simulink library "SimscapeCustomComponents_lib"  (R2025b)
settings: Solver=VariableStepAuto  StartTime=0.0  StopTime=10.0  RelTol=1e-3
undefined symbols (not defined in the file or in its folder): base, baseVdc, capacity, DiscIntNeverNeededParam, ee_sli_rtmsupport, filterInductance, freqeuncy, frequency, gcbh, gflInverter, gfmInverter, iMaxPU, Inertia, initialSOC, plantRating, solar, Ts, ups, Vac, windSystem, windTurbine
libraries: fl_lib x397, nesl_utility x171, eeGeneralControl x85, ee_lib x82, simulink x72, datacenter_lib x68, eeTransforms x38, slpidlib x24, buildingEnergy_lib x20, SimscapeFluids_lib x17, eeSinusoidalMeasurementV2 x8, eePwmGenerator x8
(part 18 of 24)

== system SimscapeCustomComponents_lib/Microgrid and Renewables/Sources/Wind Plant Integrated/Detailed/Wind Turbine and Converters/Wind Plant ==
  Pitch : Inport
  Wind speed : Inport  Port=2
  Chopper : Inport  Port=3
  Machine : Inport  Port=4
  Grid : Inport  Port=5
  Back-to-Back Converters : Subsystem  Variant=on  VariantControlMode=label  LabelModeActiveChoice=Switching  mask{converterFidelity=Switching, capDC=capDC, fSw=fSw}
      mask prompts: converterFidelity "Converter Fidelity"; capDC "DC bus capacitance (F)"; fSw "Switching Frequency (kHz)"
      settings: CopyFcn=set_param(gcb,'LinkStatus','none');
      mask TypeOptions converterFidelity: Average | Switching
      mask Callback converterFidelity: component.mask.converterFidelity(gcb);
      mask DialogControl editMSConverter Prompt: Edit machine  side converter parameters
      mask DialogControl editMSConverter Callback:
      | converterFidelity = get_param(gcb,'converterFidelity');
      | if strcmp(converterFidelity,'Average')
      |     blockPath = [gcb,'/',converterFidelity,'/','Machine Side Converter'];
      | else
      |     blockPath = [gcb,'/',converterFidelity,'/','Machine Side Converter','/','Converter'];
      | end
      |     component.mask.openConverterBlock(blockPath);
      mask DialogControl editGSConverter Prompt: Edit grid  side converter parameters
      mask DialogControl editGSConverter Callback:
      | converterFidelity = get_param(gcb,'converterFidelity');
      | if strcmp(converterFidelity,'Average')
      |     blockPath = [gcb,'/',converterFidelity,'/','Grid Side Converter'];
      | else
      |     blockPath = [gcb,'/',converterFidelity,'/','Grid Side Converter','/','Converter'];
      | end
      | component.mask.openConverterBlock(blockPath);
  Current Sensor (Three-Phase) : ee_lib/Sensors & Transducers/Current Sensor (Three-Phase)
  Ideal Torque Sensor : fl_lib/Mechanical/Mechanical Sensors/Ideal Torque Sensor
  Mechanical Rotational Reference2 : fl_lib/Mechanical/Rotational Elements/Mechanical Rotational Reference
  Mechanical Rotational Reference3 : fl_lib/Mechanical/Rotational Elements/Mechanical Rotational Reference
  PMSG : ee_lib/Electromechanical/Permanent Magnet/PMSM  port_option=ee.enum.threePhasePort.composite  winding_type=ee.enum.statorconnection.wye  machine_param=ee.enum.pmsm.parameterization.constant  nPolePairs=p  pmflux_param=ee.enum.pmflux.fluxlinkage  pm_flux_linkage=psim Wb  torque_constant=0.18 N*m/A  back_emf_constant=0.18 V*s/rad  stator_param=ee.enum.statorparam.LdLqL0  Ld=Ld H  Lq=Lq H  idVec=[-200, 0, 200] A  iqVec=[-200, 0, 200] A  LdMatrix=0.0002 * ones(3, 3) H  LqMatrix=0.0002 * ones(3, 3) H  PmMatrix=0.1 * ones(3, 3) Wb  ktMatrix=0.18 * ones(3, 3) N*m/A  keMatrix=0.18 * ones(3, 3) V*s/rad  L0=0.00016 H  Ls=0.0002 H  Lm=-0.00002 H  Ms=0.00002 H  Rs=Rs Ohm  zero_sequence=ee.enum.park.zerosequence.exclude  axes_param=ee.enum.rotorangle.qaxis  loss_param=ee.enum.ironloss.none  losses_oc=[0, 0, 0] W  losses_sc=[0, 0, 0] W  f_losses=60 Hz  Isc_losses=95 A  J=200 kg*m^2  lam=1e-2 N*m*s/rad  i_d_specify=off  i_d_priority=None  i_d=0 A  i_d_nominal_specify=off  i_d_nominal_value=1  i_d_nominal_unit=A  i_q_specify=off  i_q_priority=None  i_q=0 A  i_q_nominal_specify=off  i_q_nominal_value=1  i_q_nominal_unit=A  torque_specify=off  torque_priority=None  torque=0 N*m  torque_nominal_specify=off  torque_nominal_value=1  torque_nominal_unit=N*m  angular_velocity_specify=off  angular_velocity_priority=Low  angular_velocity=2.26 rad/s  angular_velocity_nominal_specify=off  angular_velocity_nominal_value=1  angular_velocity_nominal_unit=rpm  angular_position_specify=off  angular_position_priority=High  angular_position=0 deg  angular_position_nominal_specify=off  angular_position_nominal_value=1  angular_position_nominal_unit=deg  alpha=3.93e-3 1/K  alpha_flux=-0.001 1/K  Tmeas=298.15 K  stator_thermal_mass=100 J/K  rotor_thermal_mass=200 J/K  Rm_percent_rotor=90  Rd_percent_rotor=30  temperatureA_specify=off  temperatureA_priority=High  temperatureA=25 degC  temperatureA_nominal_specify=off  temperatureA_nominal_value=1  temperatureA_nominal_unit=degC  temperatureB_specify=off  temperatureB_priority=High  temperatureB=25 degC  temperatureB_nominal_specify=off  temperatureB_nominal_value=1  temperatureB_nominal_unit=degC  temperatureC_specify=off  temperatureC_priority=High  temperatureC=25 degC  temperatureC_nominal_specify=off  temperatureC_nominal_value=1  temperatureC_nominal_unit=degC  temperatureR_specify=off  temperatureR_priority=High  temperatureR=25 degC  temperatureR_nominal_specify=off  temperatureR_nominal_value=1  temperatureR_nominal_unit=degC
      settings: InternalSimscapePortConfiguration="{\"Bottom\":[],\"Left\":[{\"id\":\"N\",\"label\":\"~\",\"type\":\"foundation.electrical.three_phase\"}],\"Right\":[{\"id\":\"R\",\"label\":\"R\",\"type\":\"foundation.mechanical.rotational.rotational\"},{\"id\":\"C\",\"label\":\"C\",\"type\":\"foundation.mechanical.rotational.rotational\"}],\"Top\":[]}"
  PS-Simulink Converter : nesl_utility/PS-Simulink Converter  PhysicalDomain=network_engine_domain  SubClassName=ps_output  LeftPortType=input  RightPortType=output  PseudoPeriodic=off  Frequencies=[]  VectorFormat=1-D array  Unit=A  AffineConversion=off
  PS-Simulink Converter1 : nesl_utility/PS-Simulink Converter  PhysicalDomain=network_engine_domain  SubClassName=ps_output  LeftPortType=input  RightPortType=output  PseudoPeriodic=off  Frequencies=[]  VectorFormat=inherit  Unit=rad/s  AffineConversion=off
  PS-Simulink Converter5 : nesl_utility/PS-Simulink Converter  PhysicalDomain=network_engine_domain  SubClassName=ps_output  LeftPortType=input  RightPortType=output  PseudoPeriodic=off  Frequencies=[]  VectorFormat=1-D array  Unit=N*m  AffineConversion=off
  PS-Simulink Converter7 : nesl_utility/PS-Simulink Converter  PhysicalDomain=network_engine_domain  SubClassName=ps_output  LeftPortType=input  RightPortType=output  PseudoPeriodic=off  Frequencies=[]  VectorFormat=1-D array  Unit=rad  AffineConversion=off
  Rotational Motion Sensor : fl_lib/Mechanical/Mechanical Sensors/Ideal Rotational Motion Sensor  reference=foundation.enum.MeasurementReference.difference  acceleration_port=false  velocity_port=true  position_port=true  wrap_angle=simscape.enum.onoff.off  offset=0 deg
  Scope1 : Scope
      settings: ActiveDisplayYMinimum=-6255.05498425373  ActiveDisplayYMaximum=6362.825931701329  DataLoggingVariableName=ScopeData6
  Simulink-PS Converter : nesl_utility/Simulink-PS Converter  PhysicalDomain=network_engine_domain  SubClassName=ps_input  LeftPortType=input  RightPortType=output  PseudoPeriodic=off  Frequencies=[]  NoiseDistribution=none  NoiseParameters=[]  Unit=1  AffineConversion=off  FilteringAndDerivatives=provide  SimscapeFilterOrder=1  InputFilterTimeConstant=0.001  UdotUserProvided=0
  Simulink-PS Converter1 : nesl_utility/Simulink-PS Converter  PhysicalDomain=network_engine_domain  SubClassName=ps_input  LeftPortType=input  RightPortType=output  PseudoPeriodic=off  Frequencies=[]  NoiseDistribution=none  NoiseParameters=[]  Unit=1  AffineConversion=off  FilteringAndDerivatives=provide  SimscapeFilterOrder=1  InputFilterTimeConstant=0.001  UdotUserProvided=0
  Unit Delay : UnitDelay  SampleTime=-1
  Wind Turbine : ee_lib/Electromechanical/Wind Turbine (Mechanical)  R_rotor=turbineRadius m  pitch_TLU=pitch deg  lambda_TLU=TSR  Cp_TLU=cp  v_thr=wt m/s  w_thr=rt rad/s  rho_air=airDensity kg/m^3  includeInertia=false  J=Inertia kg*m^2  lam=10 N*m*s/rad  w_specify=off  w_priority=Low  w=2.262*2.5 rad/s  w_nominal_specify=off  w_nominal_value=1  w_nominal_unit=rad/s  t_specify=off  t_priority=None  t=0 N*m  t_nominal_specify=off  t_nominal_value=1  t_nominal_unit=N*m  Torque_specify=off  Torque_priority=None  Torque=0 N*m  Torque_nominal_specify=off  Torque_nominal_value=1  Torque_nominal_unit=N*m
      settings: InternalSimscapePortConfiguration="{\"Bottom\":[],\"Left\":[{\"id\":\"vWind\",\"label\":\"V\",\"type\":\"input\"},{\"id\":\"pitch\",\"label\":\"β\",\"type\":\"input\"}],\"Right\":[{\"id\":\"R\",\"label\":\"R\",\"type\":\"foundation.mechanical.rotational.rotational\"}],\"Top\":[]}"
  ~ : PMIOPort  Side=Right
  Out Bus Element2 : Outport  PortName=PMSM  Element=torque
  Out Bus Element3 : Outport  PortName=PMSM  Element=rotorSpeed
  BusElementOut : Outport  PortName=PMSM  Element=rotorAngle
  BusElementOut1 : Outport  PortName=PMSM  Element=iabc
  Out Bus Element : Outport  Port=2  PortName=Meas  Element=windSpeed
  BusElementOut2 : Outport  Port=2  PortName=Meas  Element=Vdc
  wires:
  PS-Simulink Converter7/1 -> BusElementOut/1
  Grid/1 -> Back-to-Back Converters/3(Grid_ref)
  Chopper/1 -> Back-to-Back Converters/1(Chopper)
  PS-Simulink Converter1/1 -> Out Bus Element3/1
  Pitch/1 -> Simulink-PS Converter/1
  Unit Delay/1 -> Out Bus Element/1
  PS-Simulink Converter/1 -> Scope1/1, BusElementOut1/1
  Wind speed/1 -> Unit Delay/1, Simulink-PS Converter1/1
  PS-Simulink Converter5/1 -> Out Bus Element2/1
  Machine/1 -> Back-to-Back Converters/2(SM_ref)
  Back-to-Back Converters/1(Vdc) -> BusElementOut2/1
  connections:
  Current Sensor (Three-Phase)/RConn1 -- PS-Simulink Converter/LConn1
  Back-to-Back Converters/RConn1 -- ~/RConn1
  PS-Simulink Converter7/LConn1 -- Rotational Motion Sensor/RConn3
  PS-Simulink Converter1/LConn1 -- Rotational Motion Sensor/RConn2
  Current Sensor (Three-Phase)/LConn1 -- PMSG/LConn1
  PMSG/RConn2 -- Mechanical Rotational Reference2/LConn1
  Ideal Torque Sensor/RConn1 -- Wind Turbine/RConn1 -- Rotational Motion Sensor/LConn1
  PMSG/RConn1 -- Ideal Torque Sensor/LConn1
  Mechanical Rotational Reference3/LConn1 -- Rotational Motion Sensor/RConn1
  PS-Simulink Converter5/LConn1 -- Ideal Torque Sensor/RConn2
  Current Sensor (Three-Phase)/RConn2 -- Back-to-Back Converters/LConn1
  Wind Turbine/LConn2 -- Simulink-PS Converter/RConn1
  Wind Turbine/LConn1 -- Simulink-PS Converter1/RConn1

== system SimscapeCustomComponents_lib/Microgrid and Renewables/Storage/BESS Integrated/Detailed/BESS Controller/Grid Following ==
  VRef : Inport
  FRef : Inport  Port=2
  PRef : Inport  Port=3
  QRef : Inport  Port=4
  Mode : Inport  Port=5
  Reset : Inport  Port=6
  In Bus Element3 : Inport  Port=7  PortName=VIBus  Element=Vd
  BusElementIn : Inport  Port=7  PortName=VIBus  Element=Vd
  In Bus Element2 : Inport  Port=7  PortName=VIBus  Element=Vq
  In Bus Element7 : Inport  Port=7  PortName=VIBus  Element=Theta
  BusElementIn1 : Inport  Port=7  PortName=VIBus  Element=Freq
  BusElementIn3 : Inport  Port=7  PortName=VIBus  Element=Id
  BusElementIn4 : Inport  Port=7  PortName=VIBus  Element=Iq
  Constant : Constant  Value=10
  Current_controller : Subsystem
  Inverse Park Transform1 : eeTransforms/Inverse Park Transform  AxisAlignment=Q-axis  PowerInvariant=off
  Reference Current : Subsystem
  Sum2 : Sum  Inputs=|+-
  Terminator : Terminator
  Terminator1 : Terminator
  Unit Delay : UnitDelay  SampleTime=Td
  Unit Delay1 : UnitDelay  SampleTime=Td
  Unit Delay2 : UnitDelay  SampleTime=Ts
  mabc : Outport
  wires:
  Constant/1 -> Reference Current/4(LVRT_iq)
  Reset/1 -> Terminator1/1
  Mode/1 -> Terminator/1
  In Bus Element2/1 -> Current_controller/6(Vq)
  Inverse Park Transform1/1 -> Unit Delay2/1
  Unit Delay2/1 -> mabc/1
  Current_controller/1(mdq0) -> Inverse Park Transform1/1
  In Bus Element3/1 -> Current_controller/5(Vd)
  In Bus Element7/1 -> Inverse Park Transform1/2
  FRef/1 -> Sum2/1
  VRef/1 -> Reference Current/1(V_ref)
  Sum2/1 -> Reference Current/3(del f)
  Reference Current/2(iq_ref) -> Current_controller/3(iqref)
  Reference Current/1(id_ref) -> Current_controller/1(id-ref)
  Unit Delay1/1 -> Sum2/2
  Unit Delay/1 -> Reference Current/2(V-mag)
  BusElementIn/1 -> Unit Delay/1
  BusElementIn1/1 -> Unit Delay1/1
  BusElementIn3/1 -> Current_controller/2(ipvd)
  BusElementIn4/1 -> Current_controller/4(iq)
  PRef/1 -> Reference Current/5(PRef)
  QRef/1 -> Reference Current/6(QRef)

== system SimscapeCustomComponents_lib/Microgrid and Renewables/Storage/BESS Integrated/Detailed/BESS Controller/Grid Forming ==
  VRef : Inport
  FRef : Inport  Port=2
  PRef : Inport  Port=3
  QRef : Inport  Port=4
  Mode : Inport  Port=5
  Reset : Inport  Port=6
  Bus Element In : Inport  Port=7  PortName=VIBus  Element=Vabc
  BusElementIn : Inport  Port=7  PortName=VIBus  Element=Iabc
  Current Limiting : Subsystem
  Grid Voltage Reactive Power Support : Subsystem
  Measurement : Subsystem
      mask Display: image('meas2_1_7_7_2_1.png');
  Power Control : Subsystem
  Subsystem2 : Subsystem
      settings: PortSchema="{\"entries\":[{\"content\":{\"sides\":[{\"content\":{\"connectorIds\":[\"Out1\"]},\"type\":\"ConnectorPlacement.EquallySpacedRectSide\",\"uuid\":\"7526c1f7-0aba-4355-8bbd-47d168879ecb\"},{\"content\":{\"connectorIds\":[\"In1\",\"In2\"],\"side\":\"RIGHT\"},\"type\":\"ConnectorPlacement.EquallySpacedRectSide\",\"uuid\":\"1dda9693-ec76-4df0-8ad4-aaa83d2574b3\"},{\"content\":{\"side\":\"TOP\"},\"type\":\"ConnectorPlacement.EquallySpacedRectSide\",\"uuid\":\"71ea411b-eb5f-4279-ae23-08ebb3ff1ed6\"}]},\"type\":\"ConnectorPlacement.EquallySpacedConnector\",\"uuid\":\"19864e0c-0998-460d-9705-13c69283d4ec\"}],\"packageUris\":[\"http://schema.mathworks.com/mf0/Connector/R2020b\"],\"version\":\"1.0\"}"
  Terminator : Terminator
  Terminator1 : Terminator
  Terminator2 : Terminator
  VoltageCurrentControl : Subsystem
      settings: PortSchema="{\"entries\":[{\"content\":{\"sides\":[{\"content\":{\"connectorIds\":[\"In1\",\"In2\",\"In3\"]},\"type\":\"ConnectorPlacement.EquallySpacedRectSide\",\"uuid\":\"0bf15a12-7bc0-47e4-89bd-435769673763\"},{\"content\":{\"connectorIds\":[\"Out1\"],\"side\":\"RIGHT\"},\"type\":\"ConnectorPlacement.EquallySpacedRectSide\",\"uuid\":\"44a15d74-8878-4ec6-abe4-be0b1b609519\"},{\"content\":{\"connectorIds\":[\"In4\"],\"side\":\"TOP\"},\"type\":\"ConnectorPlacement.EquallySpacedRectSide\",\"uuid\":\"7a96781e-5638-4b2a-8101-d5785aae9f0f\"}]},\"type\":\"ConnectorPlacement.EquallySpacedConnector\",\"uuid\":\"4b3373ad-cf20-4175-894e-3bd1604dd0ce\"}],\"packageUris\":[\"http://schema.mathworks.com/mf0/Connector/R2020b\"],\"version\":\"1.0\"}"
  mabc : Outport
  wires:
  Subsystem2/1(mabc) -> mabc/1
  VoltageCurrentControl/1(mabc) -> Subsystem2/1(In)
  Bus Element In/1 -> Measurement/1(Vgabcc)
  BusElementIn/1 -> Measurement/2(Igabc)
  Measurement/2(Pmeas) -> Terminator/1
  Measurement/3(Qmeas) -> Terminator1/1
  Measurement/1(measure) -> Current Limiting/1(measure), VoltageCurrentControl/4(measure), Power Control/1(measure), Grid Voltage Reactive Power Support/1(measure)
  Power Control/3(angle) -> Measurement/3(Angle)
  Power Control/1(reactiveControl) -> Current Limiting/2(reactiveControl)
  Power Control/2(activeControl) -> VoltageCurrentControl/2(activeControl)
  Current Limiting/1(currentLimiting) -> VoltageCurrentControl/1(currentLimiting)
  QRef/1 -> Grid Voltage Reactive Power Support/3(QrefInput)
  PRef/1 -> Grid Voltage Reactive Power Support/2(PrefInput)
  Grid Voltage Reactive Power Support/1(Pref) -> Power Control/2(Pref)
  Grid Voltage Reactive Power Support/2(Qref) -> Power Control/3(Qref)
  Measurement/4(fmeas) -> Terminator2/1
  FRef/1 -> Power Control/5(Fref)
  VRef/1 -> Power Control/4(Vref)
  Mode/1 -> Power Control/6(CntrlFlag)
  Reset/1 -> VoltageCurrentControl/3(Reset), Subsystem2/2(Reset)

== system SimscapeCustomComponents_lib/Microgrid and Renewables/Storage/BESS Integrated/Detailed/BESS Plant/Converter ==
  mabc : Inport
  Average : Subsystem  VariantControl=Average
  Switching : Subsystem  VariantControl=Switching
  + : PMIOPort  Side=Left
  - : PMIOPort  Port=2  Side=Left
  ~ : PMIOPort  Port=3  Side=Right

== system SimscapeCustomComponents_lib/Microgrid and Renewables/Storage/BESS Integrated/Detailed/Filter & Measurements/PLL & Measurements ==
  V : Inport
  I : Inport  Port=2
  Measurement1 : Subsystem
  Measurement2 : Subsystem
  Subsystem : Subsystem
  Out Bus Element : Outport  PortName=VIbus  Element=Vq
  Out Bus Element1 : Outport  PortName=VIbus  Element=Vd
  Out Bus Element2 : Outport  PortName=VIbus  Element=Freq
  Out Bus Element3 : Outport  PortName=VIbus  Element=Theta
  Out Bus Element4 : Outport  PortName=VIbus  Element=Vmag
  Out Bus Element5 : Outport  PortName=VIbus  Element=Iq
  Out Bus Element6 : Outport  PortName=VIbus  Element=Id
  Out Bus Element7 : Outport  PortName=VIbus  Element=Iabc
  Out Bus Element8 : Outport  PortName=VIbus  Element=Vabc
  wires:
  V/1 -> Measurement2/1(u)
  Subsystem/2(freq) -> Out Bus Element2/1
  Subsystem/5(Vq) -> Out Bus Element/1
  Subsystem/3(angle) -> Out Bus Element3/1
  Subsystem/4(Vd) -> Out Bus Element1/1
  Measurement2/1(Vg) -> Out Bus Element8/1, Subsystem/1(Vabc)
  Subsystem/1(mag) -> Out Bus Element4/1
  I/1 -> Measurement1/1(u)
  Measurement1/1(Vg) -> Out Bus Element7/1, Subsystem/2(Iabc)
  Subsystem/7(Iq1) -> Out Bus Element5/1
  Subsystem/6(Id1) -> Out Bus Element6/1

== system SimscapeCustomComponents_lib/Microgrid and Renewables/Storage/BESS Integrated/Simplified/Grid Following/Measurements ==
  Current and Voltage Sensor (Three-Phase)1 : ee_lib/Sensors & Transducers/Current and Voltage Sensor (Three-Phase)  vMeasurementType=ee.enum.vmeasurement.lg  outputUnit=ee.enum.unit.pu  SRated=plantRating*1000 A*V  VRated=Vac V  I_specify=off  I_priority=None  I=[0, 0, 0] A  I_nominal_specify=off  I_nominal_value=1  I_nominal_unit=A  V_specify=off  V_priority=None  V=[0, 0, 0] V  V_nominal_specify=off  V_nominal_value=1  V_nominal_unit=V
      settings: InternalSimscapePortConfiguration="{\"Bottom\":[],\"Left\":[{\"id\":\"N1\",\"label\":\"~1\",\"type\":\"foundation.electrical.three_phase\"}],\"Right\":[{\"id\":\"V_output\",\"label\":\"V\",\"type\":\"output\"},{\"id\":\"I_output\",\"label\":\"I\",\"type\":\"output\"},{\"id\":\"N2\",\"label\":\"~2\",\"type\":\"foundation.electrical.three_phase\"}],\"Top\":[]}"
  Gain1 : Gain  Gain=1/(plantRating*1000)
  Gain2 : Gain  Gain=1/(plantRating*1000)
  Low-Pass Filter (Discrete or Continuous)1 : eeGeneralControl/Low-Pass Filter (Discrete or Continuous)  K=1  T=0.1  B=inf  A=-inf  init_option=Inherited from block input  x0=0  Ts=-1
  Low-Pass Filter (Discrete or Continuous)2 : eeGeneralControl/Low-Pass Filter (Discrete or Continuous)  K=1  T=0.1  B=inf  A=-inf  init_option=Inherited from block input  x0=0  Ts=-1
  PS-Simulink Converter{,1..3} (4 alike) : nesl_utility/PS-Simulink Converter  PhysicalDomain=network_engine_domain  SubClassName=ps_output  LeftPortType=input  RightPortType=output  PseudoPeriodic=off  Frequencies=[]  VectorFormat=inherit  Unit=inherit  AffineConversion=off
  Power Sensor (Three-Phase) : ee_lib/Sensors & Transducers/Power Sensor (Three-Phase)  load_type=ee.enum.passive.type_balanced.balanced  f0=60 Hz
      settings: InternalSimscapePortConfiguration="{\"Bottom\":[],\"Left\":[{\"id\":\"N1\",\"label\":\"~1\",\"type\":\"foundation.electrical.three_phase\"}],\"Right\":[{\"id\":\"N2\",\"label\":\"~2\",\"type\":\"foundation.electrical.three_phase\"}],\"Top\":[{\"id\":\"Pm\",\"label\":\"P\",\"type\":\"output\"},{\"id\":\"Qm\",\"label\":\"Q\",\"type\":\"output\"}]}"
  In : PMIOPort  Side=Left
  ~ : PMIOPort  Port=2  Side=Right
  P : Outport
  Q : Outport  Port=2
  V : Outport  Port=3
  I : Outport  Port=4
  wires:
  PS-Simulink Converter/1 -> Low-Pass Filter (Discrete or Continuous)1/1
  PS-Simulink Converter1/1 -> Low-Pass Filter (Discrete or Continuous)2/1
  Low-Pass Filter (Discrete or Continuous)1/1 -> Gain1/1
  Low-Pass Filter (Discrete or Continuous)2/1 -> Gain2/1
  PS-Simulink Converter2/1 -> V/1
  PS-Simulink Converter3/1 -> I/1
  Gain1/1 -> P/1
  Gain2/1 -> Q/1
  connections:
  Current and Voltage Sensor (Three-Phase)1/RConn1 -- PS-Simulink Converter2/LConn1
  PS-Simulink Converter/LConn1 -- Power Sensor (Three-Phase)/LConn2
  In/RConn1 -- Power Sensor (Three-Phase)/LConn1
  Current and Voltage Sensor (Three-Phase)1/RConn3 -- ~/RConn1
  PS-Simulink Converter1/LConn1 -- Power Sensor (Three-Phase)/LConn3
  Current and Voltage Sensor (Three-Phase)1/LConn1 -- Power Sensor (Three-Phase)/RConn1
  Current and Voltage Sensor (Three-Phase)1/RConn2 -- PS-Simulink Converter3/LConn1

== system SimscapeCustomComponents_lib/Microgrid and Renewables/Storage/BESS Integrated/Simplified/Grid Following/Power Limiter ==
  P : Inport
  SOC : Inport  Port=2
  V : Inport  Port=3
  Add : Sum
  Compare To Constant : simulink/Logic and Bit Operations/Compare To Constant  relop=<=  const=minSOC  OutDataTypeStr=boolean
  Compare To Constant1 : simulink/Logic and Bit Operations/Compare To Constant  relop=>=  const=maxSOC  OutDataTypeStr=boolean
  Constant : Constant  Value=maxSOC
  Constant1 : Constant  Value=0
  Constant2 : Constant  Value=minSOC
  Constant3 : Constant  Value=0
  Constant5 : Constant  Value=minSOC
  Data Type Conversion : DataTypeConversion  OutDataTypeStr=double  SaturateOnIntegerOverflow=off  RndMeth=Floor
  Delay1 : Delay  DelayLength=1
  Divide : Product  Inputs=*/
  Gain : Gain  Gain=-1/(Inf)
  GreaterThan : RelationalOperator  Operator=>  OutDataTypeStr=boolean  RndMeth=Simplest  InputSameDT=off
  GreaterThan1 : RelationalOperator  Operator=<  OutDataTypeStr=boolean  RndMeth=Simplest  InputSameDT=off
  GreaterThan3 : RelationalOperator  Operator=<  OutDataTypeStr=boolean  RndMeth=Simplest  InputSameDT=off
  NOR : Logic  Operator=NOR  IconShape=distinctive  AllPortsSameDT=off  OutDataTypeStr=boolean
  Product : Product
  Scope1 : Scope  NumInputPorts=2
  Scope2 : Scope
  Scope3 : Scope  NumInputPorts=3
  Switch : Switch  Criteria=u2 > Threshold  SaturateOnIntegerOverflow=off  InputSameDT=off
  Switch1 : Switch  Criteria=u2 > Threshold  SaturateOnIntegerOverflow=off  InputSameDT=off
  Switch2 : Switch  Criteria=u2 > Threshold  SaturateOnIntegerOverflow=off  InputSameDT=off
  POut : Outport
  SOCFlag : Outport  Port=2
  wires:
  P/1 -> Scope3/2, Switch2/2, Switch1/3, Switch/3
  Switch1/1 -> Scope3/1, Switch2/1
  Constant3/1 -> Switch1/1
  GreaterThan1/1 -> Scope1/1, Switch1/2
  Constant2/1 -> GreaterThan1/2
  Constant1/1 -> Switch/1
  GreaterThan/1 -> Switch/2
  Constant/1 -> GreaterThan/2
  Constant5/1 -> GreaterThan3/2
  GreaterThan3/1 -> SOCFlag/1
  V/1 -> Delay1/1
  Delay1/1 -> Divide/2
  Divide/1 -> Gain/1
  SOC/1 -> Add/2, GreaterThan3/1, Scope2/1, GreaterThan1/1, GreaterThan/1
  Switch/1 -> Scope3/3, Switch2/3
  Switch2/1 -> Divide/1, Product/1
  Add/1 -> Compare To Constant/1, Compare To Constant1/1
  Compare To Constant/1 -> NOR/1
  Compare To Constant1/1 -> NOR/2
  NOR/1 -> Data Type Conversion/1
  Data Type Conversion/1 -> Product/2
  Gain/1 -> Add/1
  Product/1 -> POut/1

== system SimscapeCustomComponents_lib/Microgrid and Renewables/Storage/BESS Integrated/Simplified/Grid Following/SOC Estimation ==
  I : Inport
  Constant : Constant  Value=0.95
  Gain : Gain  Gain=-1/(100000)
  Integrator (Discrete or Continuous) : eeGeneralControl/Integrator (Discrete or Continuous)  LabelModeActiveChoice=Discrete  IntegratorMethod=Integration: Forward Euler  ExternalReset=level  LimitType=Anti-windup  B=inf  A=-inf  Ts=-1
  SOC : Outport
  wires:
  Constant/1 -> Integrator (Discrete or Continuous)/3
  I/1 -> Gain/1
  Gain/1 -> Integrator (Discrete or Continuous)/1
  Integrator (Discrete or Continuous)/1 -> SOC/1

== system SimscapeCustomComponents_lib/Microgrid and Renewables/Storage/BESS Integrated/Simplified/Grid Forming/Limiter ==
  SOC : Inport
  Compare To Constant : simulink/Logic and Bit Operations/Compare To Constant  relop=<=  const=minSOC  OutDataTypeStr=boolean
  Compare To Constant1 : simulink/Logic and Bit Operations/Compare To Constant  relop=>=  const=maxSOC  OutDataTypeStr=boolean
  Data Type Conversion : DataTypeConversion  OutDataTypeStr=double  SaturateOnIntegerOverflow=off  RndMeth=Floor
  Delay : Delay  DelayLength=1  InputProcessing=Columns as channels (frame based)
  OR : Logic  Operator=OR  AllPortsSameDT=off  OutDataTypeStr=boolean
  Flag : Outport
  wires:
  SOC/1 -> Compare To Constant/1, Compare To Constant1/1
  Compare To Constant/1 -> OR/1
  Compare To Constant1/1 -> OR/2
  OR/1 -> Data Type Conversion/1
  Data Type Conversion/1 -> Delay/1
  Delay/1 -> Flag/1

== system SimscapeCustomComponents_lib/Microgrid and Renewables/Storage/BESS Integrated/Simplified/Grid Forming/Measurements ==
  Current and Voltage Sensor (Three-Phase)1 : ee_lib/Sensors & Transducers/Current and Voltage Sensor (Three-Phase)  vMeasurementType=ee.enum.vmeasurement.lg  outputUnit=ee.enum.unit.pu  SRated=plantRating*1000 A*V  VRated=Vac V  I_specify=off  I_priority=None  I=[0, 0, 0] A  I_nominal_specify=off  I_nominal_value=1  I_nominal_unit=A  V_specify=off  V_priority=None  V=[0, 0, 0] V  V_nominal_specify=off  V_nominal_value=1  V_nominal_unit=V
      settings: InternalSimscapePortConfiguration="{\"Bottom\":[],\"Left\":[{\"id\":\"N1\",\"label\":\"~1\",\"type\":\"foundation.electrical.three_phase\"}],\"Right\":[{\"id\":\"V_output\",\"label\":\"V\",\"type\":\"output\"},{\"id\":\"I_output\",\"label\":\"I\",\"type\":\"output\"},{\"id\":\"N2\",\"label\":\"~2\",\"type\":\"foundation.electrical.three_phase\"}],\"Top\":[]}"
  Gain1 : Gain  Gain=1/(plantRating*1000)
  Gain2 : Gain  Gain=1/(plantRating*1000)
  PS-Simulink Converter{,1..3} (4 alike) : nesl_utility/PS-Simulink Converter  PhysicalDomain=network_engine_domain  SubClassName=ps_output  LeftPortType=input  RightPortType=output  PseudoPeriodic=off  Frequencies=[]  VectorFormat=inherit  Unit=inherit  AffineConversion=off
  Power Sensor (Three-Phase) : ee_lib/Sensors & Transducers/Power Sensor (Three-Phase)  load_type=ee.enum.passive.type_balanced.balanced  f0=60 Hz
      settings: InternalSimscapePortConfiguration="{\"Bottom\":[],\"Left\":[{\"id\":\"N1\",\"label\":\"~1\",\"type\":\"foundation.electrical.three_phase\"}],\"Right\":[{\"id\":\"N2\",\"label\":\"~2\",\"type\":\"foundation.electrical.three_phase\"}],\"Top\":[{\"id\":\"Pm\",\"label\":\"P\",\"type\":\"output\"},{\"id\":\"Qm\",\"label\":\"Q\",\"type\":\"output\"}]}"
  In : PMIOPort  Side=Left
  ~ : PMIOPort  Port=2  Side=Right
  P : Outport
  Q : Outport  Port=2
  V : Outport  Port=3
  I : Outport  Port=4
  wires:
  Gain2/1 -> Q/1
  Gain1/1 -> P/1
  PS-Simulink Converter3/1 -> I/1
  PS-Simulink Converter2/1 -> V/1
  PS-Simulink Converter/1 -> Gain1/1
  PS-Simulink Converter1/1 -> Gain2/1
  connections:
  Current and Voltage Sensor (Three-Phase)1/RConn2 -- PS-Simulink Converter3/LConn1
  Current and Voltage Sensor (Three-Phase)1/LConn1 -- Power Sensor (Three-Phase)/RConn1
  PS-Simulink Converter1/LConn1 -- Power Sensor (Three-Phase)/LConn3
  Current and Voltage Sensor (Three-Phase)1/RConn3 -- ~/RConn1
  In/RConn1 -- Power Sensor (Three-Phase)/LConn1
  PS-Simulink Converter/LConn1 -- Power Sensor (Three-Phase)/LConn2
  Current and Voltage Sensor (Three-Phase)1/RConn1 -- PS-Simulink Converter2/LConn1

== system SimscapeCustomComponents_lib/Microgrid and Renewables/Storage/BESS Integrated/Simplified/Grid Forming/Reference Generator ==
  Mode : Inport
  PRef : Inport  Port=2
  P : Inport  Port=3
  QRef : Inport  Port=4
  Q : Inport  Port=5
  VRef : Inport  Port=6
  V : Inport  Port=7
  Gain : Gain  Gain=efficiency/100
  Gain2 : Gain  Gain=sqrt(3)/Vac
  If : If
  If Action Subsystem : Subsystem  TreatAsAtomicUnit=on
  If Action Subsystem1 : Subsystem  TreatAsAtomicUnit=on
  Merge : Merge
  Merge1 : Merge
  Vt : Outport
  Ph : Outport  Port=2
  wires:
  Merge/1 -> Vt/1
  Gain2/1 -> If Action Subsystem1/4(V)
  Q/1 -> If Action Subsystem/4(Q)
  P/1 -> If Action Subsystem1/2(P), If Action Subsystem/2(P)
  Merge1/1 -> Ph/1
  If Action Subsystem1/2(Ph) -> Merge1/2
  If Action Subsystem/2(Ph) -> Merge1/1
  If Action Subsystem1/1(Vt) -> Merge/2
  If Action Subsystem/1(Vt) -> Merge/1
  If/2 -> If Action Subsystem1/Action
  V/1 -> Gain2/1
  VRef/1 -> If Action Subsystem1/3(VRef)
  QRef/1 -> If Action Subsystem/3(QRef)
  PRef/1 -> If Action Subsystem1/1(PRef), Gain/1
  If/1 -> If Action Subsystem/Action
  Mode/1 -> If/1
  Gain/1 -> If Action Subsystem/1(PRef)

== system SimscapeCustomComponents_lib/Microgrid and Renewables/Storage/BESS Integrated/Simplified/Grid Forming/SOC Estimation ==
  P : Inport
  Constant : Constant  Value=Vdc
  Constant1 : Constant  Value=initialSOC
  Constant2 : Constant  Value=capacity
  Constant3 : Constant  Value=Inf
  Divide : Product  Inputs=*/
  Divide1 : Product  Inputs=*/
  Gain : Gain  Gain=-plantRating*1000
  Integrator (Discrete or Continuous) : eeGeneralControl/Integrator (Discrete or Continuous)  LabelModeActiveChoice=Discrete  IntegratorMethod=Integration: Forward Euler  ExternalReset=level  LimitType=Anti-windup  B=inf  A=-inf  Ts=-1
  String Compare : StringCompare
  String Constant : StringConstant  String=capacityType
  String Constant1 : StringConstant  String="\"Fixed\""
  Switch : Switch  Criteria=u2 > Threshold  SaturateOnIntegerOverflow=off  InputSameDT=off
  Meas : Outport
  wires:
  Constant3/1 -> Switch/3
  Constant2/1 -> Switch/1
  Divide1/1 -> Integrator (Discrete or Continuous)/1
  Switch/1 -> Divide1/2
  String Compare/1 -> Switch/2
  String Constant1/1 -> String Compare/2
  String Constant/1 -> String Compare/1
  Integrator (Discrete or Continuous)/1 -> Meas/1
  Constant1/1 -> Integrator (Discrete or Continuous)/3
  Divide/1 -> Divide1/1
  Constant/1 -> Divide/2
  P/1 -> Gain/1
  Gain/1 -> Divide/1

== system SimscapeCustomComponents_lib/Microgrid and Renewables/Storage/BESS Plant/Converter/Switching/Pulse Generation ==
  G : Inport
  Constant : Constant  Value=5
  Subtract : Sum  Inputs=-+
  G1 : Outport  VectorParamsAs1DForOutWhenUnconnected=off
  G2 : Outport  Port=2  VectorParamsAs1DForOutWhenUnconnected=off
  wires:
  Subtract/1 -> G2/1
  Constant/1 -> Subtract/2
  G/1 -> G1/1, Subtract/1

== system SimscapeCustomComponents_lib/Datacenter/Facilities/Solid State Transformer/PFC Rectifier Controller/Current Controller/Id and Iq Controller/Id Reference Selector ==
  Vmag : Inport
  AND1 : Logic  IconShape=distinctive  AllPortsSameDT=off  OutDataTypeStr=boolean
  Bias : Bias  Bias=0.01  SaturateOnIntegerOverflow=off
  Compare To Constant : simulink/Logic and Bit Operations/Compare To Constant  relop=>  const=0.5  OutDataTypeStr=boolean
  Compare To Constant2 : simulink/Logic and Bit Operations/Compare To Constant  relop=>  const=0.05  OutDataTypeStr=boolean
  Data Type Conversion : DataTypeConversion  SaturateOnIntegerOverflow=off  RndMeth=Floor
  Data Type Conversion1 : DataTypeConversion  OutDataTypeStr=double  SaturateOnIntegerOverflow=off  RndMeth=Floor
  Discrete-Time Integrator : DiscreteIntegrator  IntegratorMethod=Integration: Backward Euler  ExternalReset=falling  SampleTime=ups.sampleTime  LimitOutput=on  UpperSaturationLimit=0.6  LowerSaturationLimit=0  ICPrevOutput=DiscIntNeverNeededParam  ICPrevScaledInput=DiscIntNeverNeededParam
  Mode : Outport
  wires:
  Data Type Conversion/1 -> Mode/1
  Data Type Conversion1/1 -> Discrete-Time Integrator/2, Discrete-Time Integrator/1, AND1/1
  Discrete-Time Integrator/1 -> Compare To Constant2/1
  Compare To Constant2/1 -> AND1/2
  AND1/1 -> Data Type Conversion/1
  Compare To Constant/1 -> Data Type Conversion1/1
  Vmag/1 -> Bias/1
  Bias/1 -> Compare To Constant/1

== system SimscapeCustomComponents_lib/Datacenter/Facilities/Solid State Transformer/PFC Rectifier Controller/DC Voltage Controller and Current Reference/Voltage Controller/Voltage control ==
  e : Inport
  Reset : Inport  Port=2
  Discrete-Time Integrator : DiscreteIntegrator  IntegratorMethod=Integration: Backward Euler  ExternalReset=falling  SampleTime=ups.sampleTime  LimitOutput=on  UpperSaturationLimit=1  LowerSaturationLimit=0  ICPrevOutput=DiscIntNeverNeededParam  ICPrevScaledInput=DiscIntNeverNeededParam
  Ki : Gain  Gain=KiVoltage
  Kp : Gain  Gain=KpVoltage
  Sum7 : Sum  Inputs=|++
  u : Outport  VectorParamsAs1DForOutWhenUnconnected=off
  wires:
  e/1 -> Ki/1, Kp/1
  Ki/1 -> Discrete-Time Integrator/1
  Sum7/1 -> u/1
  Kp/1 -> Sum7/1
  Discrete-Time Integrator/1 -> Sum7/2
  Reset/1 -> Discrete-Time Integrator/2

== system SimscapeCustomComponents_lib/Microgrid and Renewables/Control/BESS/Grid Forming Control/Current Limiting/CurrentLimitingMethod/currentLimitAndVirtual ==
  Igd : Inport
  Igq : Inport  Port=2
  Current Saturation : Subsystem
  CurrentLimitSelection : Stateflow chart  TreatAsAtomicUnit=on
  Math Function : Math  Operator=hypot
  Merge{,1..3} (4 alike) : Merge  Inputs=3
  No Fault Ride Through : Subsystem
  VI : Subsystem
  delVd : Outport
  delVq : Outport  Port=2
  Idmax : Outport  Port=3
  Iqmax : Outport  Port=4
  wires:
  Merge2/1 -> Idmax/1
  Igq/1 -> Current Saturation/2(Iq), VI/2(Iq), No Fault Ride Through/2(Iq), [Iq]
  Merge1/1 -> delVq/1
  Igd/1 -> VI/1(Id), Current Saturation/1(Id), No Fault Ride Through/1(Id), [Id]
  No Fault Ride Through/1(delVd) -> Merge/3
  No Fault Ride Through/3(idmax) -> Merge2/3
  VI/1(delVd) -> Merge/1
  [Iq] -> Math Function/2
  [Id] -> Math Function/1
  Current Saturation/1(delVd) -> Merge/2
  Current Saturation/4(iqmax) -> Merge3/2
  Merge/1 -> delVd/1
  VI/2(delVq) -> Merge1/1
  Current Saturation/3(idmax) -> Merge2/2
  VI/4(iqmax) -> Merge3/1
  VI/3(idmax) -> Merge2/1
  No Fault Ride Through/4(iqmax) -> Merge3/3
  Current Saturation/2(delVq) -> Merge1/2
  Merge3/1 -> Iqmax/1
  No Fault Ride Through/2(delVq) -> Merge1/3
  Math Function/1 -> CurrentLimitSelection/1(Is)
  CurrentLimitSelection/1(ismax) -> [Imax]
  CurrentLimitSelection/2(noCurrentLimit) -> [noCtLt]
  CurrentLimitSelection/3(viCurrentLimit) -> [viCtLt]
  CurrentLimitSelection/4(satCurrentLimit) -> [satCtLt]
  [viCtLt] -> VI/Enable
  [satCtLt] -> Current Saturation/Enable
  [noCtLt] -> No Fault Ride Through/Enable
  [Imax] -> Current Saturation/3(Imaxsat)
  [Imax] -> VI/3(Imax)

== system SimscapeCustomComponents_lib/Microgrid and Renewables/Control/BESS/Grid Forming Control/Current Limiting/CurrentLimitingMethod/currentSaturation ==
  note: Vs-delV
  Igd : Inport
  Igq : Inport  Port=2
  Compare : Subsystem
  Constant : Constant  Value=maxSatCurrentLimit
  Constant1 : Constant  Value=0
  Constant2 : Constant  Value=0
  If : If
  If Action Subsystem : Subsystem  TreatAsAtomicUnit=on
  If Action Subsystem1 : Subsystem  TreatAsAtomicUnit=on
  Math Function : Math  Operator=hypot
  Merge : Merge
  Merge1 : Merge
  Subtract : Sum  Inputs=+-
  delVd : Outport
  delVq : Outport  Port=2
  Idmax : Outport  Port=3
  Iqmax : Outport  Port=4
  wires:
  Igd/1 -> [Isd], Math Function/1
  Igq/1 -> [Isq], Math Function/2
  Constant/1 -> Subtract/1
  Math Function/1 -> [Is], Subtract/2  "Is"
  If/1 -> If Action Subsystem/Action
  [Isd] -> If Action Subsystem/2(Isd)
  [Isq] -> If Action Subsystem/3(Isq)
  Subtract/1 -> Compare/1(u)
  Compare/1(Out1) -> If/1
  If/2 -> If Action Subsystem1/Action
  [Is] -> If Action Subsystem/1(Is)
  If Action Subsystem/1(Idmax) -> Merge/1
  If Action Subsystem1/1(Idmax) -> Merge/2
  If Action Subsystem/2(Iqmax) -> Merge1/1
  If Action Subsystem1/2(Iqmax) -> Merge1/2
  Constant2/1 -> delVq/1
  Constant1/1 -> delVd/1
  Merge/1 -> Idmax/1
  Merge1/1 -> Iqmax/1

== system SimscapeCustomComponents_lib/Microgrid and Renewables/Control/BESS/Grid Forming Control/Current Limiting/CurrentLimitingMethod/virtualImpedance ==
  note: X/R ratio
  note: Resistance coefficient
  Igd : Inport
  Igq : Inport  Port=2
  Constant : Constant  Value=maxVICurrentLimit
  Constant1 : Constant  Value=0
  Constant2 : Constant  Value=0
  Constant3 : Constant  Value=0
  Gain : Gain  Gain=ctLimitVirtualImp
  Gain1 : Gain  Gain=ctLimitXbyR
  Low-Pass Filter : eeGeneralControl/Low-Pass Filter (Discrete or Continuous)  K=1  T=currentVITimeConst  B=inf  A=-inf  init_option=Inherited from block input  x0=0  Ts=-1
  Math Function : Math  Operator=hypot
  Product{,1..3} (4 alike) : Product
  Relay : Relay  OnSwitchValue=0.01  OffSwitchValue=-0.05
  Saturation : Saturate  UpperLimit=1  LowerLimit=-1
  Saturation1 : Saturate  UpperLimit=1  LowerLimit=-1
  Sum : Sum  Inputs=|+-
  Sum1 : Sum  Inputs=|+-
  Sum2 : Sum  Inputs=++|
  Switch : Switch  Criteria=u2 > Threshold  SaturateOnIntegerOverflow=off  InputSameDT=off
  delVd : Outport
  delVq : Outport  Port=2
  Idmax : Outport  Port=3
  Iqmax : Outport  Port=4
  wires:
  Sum/1 -> Gain/1, Relay/1
  Igq/1 -> [Igq], Math Function/2
  Product1/1 -> Sum2/1
  Gain1/1 -> Product1/2, Product2/1
  Sum1/1 -> Saturation/1
  Product/1 -> Sum1/1
  Product2/1 -> Sum1/2
  Constant/1 -> Sum/2  "IsMaxium"
  Math Function/1 -> Low-Pass Filter/1  "Is"
  [Igq] -> Product3/1, Product2/2
  Switch/1 -> Gain1/1, Product3/2, Product/1
  [Igd] -> Product1/1, Product/2
  Constant2/1 -> Idmax/1
  Constant3/1 -> Iqmax/1
  Gain/1 -> Switch/1
  Constant1/1 -> Switch/3
  Igd/1 -> Math Function/1, [Igd]
  Saturation1/1 -> delVq/1
  Relay/1 -> Switch/2
  Saturation/1 -> delVd/1
  Low-Pass Filter/1 -> Sum/1
  Product3/1 -> Sum2/2
  Sum2/1 -> Saturation1/1

== system SimscapeCustomComponents_lib/Microgrid and Renewables/Control/BESS/Grid Forming Control/Grid Voltage Reactive Power Support/Modifying Active Power Reference/Computing New Active Power Ref ==
  Iq : Inport
  Vd : Inport  Port=2
  Abs : Abs  SaturateOnIntegerOverflow=off
  Constant : Constant  Value=maxVICurrentLimit*0.96
  Constant1 : Constant  Value=0
  Product : Product
  Sqrt : Sqrt
  Square : Math  Operator=square
  Square1 : Math  Operator=square
  Subtract : Sum  Inputs=-+
  Switch : Switch  Criteria=u2 > Threshold  Threshold=1.15  SaturateOnIntegerOverflow=off  InputSameDT=off
  Pref : Outport
  wires:
  Abs/1 -> Switch/3
  Constant/1 -> Square1/1
  Subtract/1 -> Sqrt/1
  Switch/1 -> Product/2
  Square/1 -> Subtract/1, Switch/2
  Square1/1 -> Subtract/2
  Constant1/1 -> Switch/1
  Vd/1 -> Product/1
  Sqrt/1 -> Abs/1
  Iq/1 -> Square/1
  Product/1 -> Pref/1

== system SimscapeCustomComponents_lib/Microgrid and Renewables/Control/BESS/Grid Forming Control/Grid Voltage Reactive Power Support/Modifying Reactive Power Reference/Changing the Power Reference ==
  Vs : Inport
  Vd : Inport  Port=2
  Pref : Inport  Port=3
  Qref : Inport  Port=4
  Enable : EnablePort
  ActivePowerReference : Subsystem
  Constant1 : Constant  Value=voltreference*0.96
  EstimateIdForGivenIq : Subsystem
  EstimateIqForReactivePower : Subsystem
  Max : MinMax  Function=max  Inputs=2
  ReactivePowerReference : Subsystem
  Prefv : Outport
  Qrefv : Outport  Port=2
  wires:
  ActivePowerReference/1(PrefNew) -> Prefv/1
  Max/1 -> Qrefv/1
  EstimateIqForReactivePower/1(Iq) -> EstimateIdForGivenIq/1(Iq), ReactivePowerReference/2(Iq)
  Constant1/1 -> EstimateIqForReactivePower/1(Vmin)
  Vs/1 -> ActivePowerReference/2(Vd), EstimateIqForReactivePower/3(Vs), ReactivePowerReference/1(Vd)
  EstimateIdForGivenIq/1(Id) -> ActivePowerReference/1(Id)
  Pref/1 -> ActivePowerReference/3(Pref)
  ReactivePowerReference/1(QrefNew) -> Max/1
  Qref/1 -> Max/2
  Vd/1 -> EstimateIqForReactivePower/2(Vd)

== system SimscapeCustomComponents_lib/Microgrid and Renewables/Control/BESS/Grid Forming Control/Grid Voltage Reactive Power Support/Modifying Reactive Power Reference/Hysteresis ==
  Vs : Inport
  AND : Logic  IconShape=distinctive  AllPortsSameDT=off  OutDataTypeStr=boolean
  Compare To Constant : simulink/Logic and Bit Operations/Compare To Constant  relop=<  const=0.9  OutDataTypeStr=boolean
  Compare To Constant1 : simulink/Logic and Bit Operations/Compare To Constant  relop=<  const=0.95  OutDataTypeStr=boolean
  D Latch : simulink_extras/Flip Flops/D Latch
  OR : Logic  Operator=OR  IconShape=distinctive  AllPortsSameDT=off  OutDataTypeStr=boolean
  Scope : Scope
      settings: ActiveDisplayYMinimum=0.96929  ActiveDisplayYMaximum=1.01111
  Terminator : Terminator
  LVFlag : Outport
  wires:
  Compare To Constant1/1 -> AND/1
  D Latch/1 -> AND/2
  AND/1 -> OR/1
  OR/1 -> LVFlag/1
  D Latch/2 -> Terminator/1
  Compare To Constant/1 -> D Latch/1, D Latch/2, OR/2
  Vs/1 -> Scope/1, Compare To Constant1/1, Compare To Constant/1

== system SimscapeCustomComponents_lib/Microgrid and Renewables/Control/BESS/Grid Forming Control/Grid Voltage Reactive Power Support/Modifying Reactive Power Reference/Not Altering the Power Reference ==
  Pref : Inport
  Qref : Inport  Port=2
  Enable : EnablePort
  Prefv : Outport
  Qrefv : Outport  Port=2
  wires:
  Pref/1 -> Prefv/1
  Qref/1 -> Qrefv/1

== system SimscapeCustomComponents_lib/Microgrid and Renewables/Control/BESS/Grid Forming Control/Measurement/Frequency Measurement/Frequency Measurement ==
  abc : Inport
  Constant : Constant
  Discrete-Time Integrator : DiscreteIntegrator  SampleTime=sampleTime  LimitOutput=on  ICPrevOutput=DiscIntNeverNeededParam  ICPrevScaledInput=DiscIntNeverNeededParam
  If : If  IfExpression=u1 > 0.9
  If Action Subsystem : Subsystem  TreatAsAtomicUnit=on
  If Action Subsystem1 : Subsystem  TreatAsAtomicUnit=on
  Merge : Merge
  Postive Sequence : Subsystem
  Freq : Outport
  wires:
  If/1 -> If Action Subsystem/Action
  If/2 -> If Action Subsystem1/Action
  Discrete-Time Integrator/1 -> If Action Subsystem/2(Time), If/1
  abc/1 -> Postive Sequence/1(abc)
  Constant/1 -> Discrete-Time Integrator/1
  If Action Subsystem/1(Freq) -> Merge/1
  If Action Subsystem1/1(Out1) -> Merge/2
  Merge/1 -> Freq/1
  Postive Sequence/1(posSeq) -> If Action Subsystem/1(V)

== system SimscapeCustomComponents_lib/Microgrid and Renewables/Control/BESS/Grid Forming Control/Measurement/abc2dq/Supply Current to dq ==
  abc : Inport
  Angle : Inport  Port=2
  Demux : Demux  Outputs=3
  Park Transform : eeTransforms/Park Transform  AxisAlignment=D-axis  PowerInvariant=off
  Terminator : Terminator
  Igd : Outport  VectorParamsAs1DForOutWhenUnconnected=off
  Igq : Outport  Port=2  VectorParamsAs1DForOutWhenUnconnected=off
  wires:
  Demux/3 -> Terminator/1
  Park Transform/1 -> Demux/1
  Demux/2 -> Igq/1
  Demux/1 -> Igd/1
  abc/1 -> Park Transform/1
  Angle/1 -> Park Transform/2

== system SimscapeCustomComponents_lib/Microgrid and Renewables/Control/BESS/Grid Forming Control/Measurement/abc2dq/Supply Voltage  to dq1 ==
  Angle : Inport
  abc : Inport  Port=2
  Demux : Demux  Outputs=3
  Park Transform : eeTransforms/Park Transform  AxisAlignment=D-axis  PowerInvariant=off
  Terminator : Terminator
  Vgd : Outport  VectorParamsAs1DForOutWhenUnconnected=off
  Vgq : Outport  Port=2  VectorParamsAs1DForOutWhenUnconnected=off
  wires:
  Demux/3 -> Terminator/1
  Park Transform/1 -> Demux/1
  Demux/2 -> Vgq/1
  Demux/1 -> Vgd/1
  abc/1 -> Park Transform/1
  Angle/1 -> Park Transform/2

== system SimscapeCustomComponents_lib/Microgrid and Renewables/Control/BESS/Grid Forming Control/Power Control/ActivePowerControl/droopControl ==
  Pref : Inport
  Pmeas : Inport  Port=2
  fref : Inport  Port=3
  cntrlflag : Inport  Port=4
  fgrid : Inport  Port=5
  Add : Sum  Inputs=+-
  Constant : Constant
  Constant5 : Constant  Value=pi/2
  Gain : Gain  Gain=powerFreq*2*pi
  Integrator with Wrapped State (Discrete or Continuous) : eeGeneralControl/Integrator with Wrapped State (Discrete or Continuous)  LabelModeActiveChoice=Discrete  WrappedStateUpperValue=2*pi  WrappedStateLowerValue=0  x0=0  Ts=activePowerSampleTime
  Lead-Lag (Discrete or Continuous) : eeGeneralControl/Lead-Lag (Discrete or Continuous)  T1=droopT1  T2=droopT2  B=inf  A=-inf  init_option=Inherited from block input  x0=0  Ts=activePowerSampleTime
  Low-Pass Filter (Discrete or Continuous) : eeGeneralControl/Low-Pass Filter (Discrete or Continuous)  K=1  T=droopTC  B=inf  A=-inf  init_option=Specify as parameter  x0=0  Ts=activePowerSampleTime
  Scope : Scope
  Scope1 : Scope
  Scope2 : Scope
  Sum : Sum  Inputs=|-+
  Sum1 : Sum  Inputs=|-+
  Terminator : Terminator
  Terminator1 : Terminator
  Terminator2 : Terminator
  mp : Gain  Gain=droopSlope
  Theta : Outport
  w : Outport  Port=2
  wires:
  Low-Pass Filter (Discrete or Continuous)/1 -> Scope2/1, Sum1/1
  mp/1 -> Low-Pass Filter (Discrete or Continuous)/1
  Sum/1 -> Scope/1, mp/1
  Pmeas/1 -> Lead-Lag (Discrete or Continuous)/1
  Add/1 -> Scope1/1, Theta/1
  Constant5/1 -> Add/2
  Pref/1 -> Sum/1
  Gain/1 -> Integrator with Wrapped State (Discrete or Continuous)/1, w/1
  Lead-Lag (Discrete or Continuous)/1 -> Sum/2
  Integrator with Wrapped State (Discrete or Continuous)/1 -> Add/1
  Constant/1 -> Sum1/2
  Sum1/1 -> Gain/1
  fgrid/1 -> Terminator/1
  fref/1 -> Terminator1/1
  cntrlflag/1 -> Terminator2/1

== system SimscapeCustomComponents_lib/Microgrid and Renewables/Control/BESS/Grid Forming Control/Power Control/ActivePowerControl/vsmControl ==
  note: Measured power
  note: Damping power input
  Pref : Inport
  Pmeas : Inport  Port=2
  fref : Inport  Port=3
  cntrlflag : Inport  Port=4
  fgrid : Inport  Port=5
  Add : Sum  Inputs=+-
  Constant2 : Constant  Value=pi/2
  Damping Frequency : Subsystem  Variant=on  VariantControlMode=label  VariantControl=Choice  LabelModeActiveChoice=constFreq
  Discrete-Time Integrator : DiscreteIntegrator  IntegratorMethod=Integration: Backward Euler  InitialCondition=1  SampleTime=activePowerSampleTime  LimitOutput=on  UpperSaturationLimit=1.1  LowerSaturationLimit=0.9  ICPrevOutput=DiscIntNeverNeededParam  ICPrevScaledInput=DiscIntNeverNeededParam
  Gain : Gain  Gain=powerFreq*2*pi
  Gain1 : Gain  Gain=1/vsmInertiaTC
  Gain2 : Gain  Gain=vsmDampingConst*powerFreq
  Integrator with Wrapped State (Discrete or Continuous) : eeGeneralControl/Integrator with Wrapped State (Discrete or Continuous)  LabelModeActiveChoice=Discrete  WrappedStateUpperValue=2*pi  WrappedStateLowerValue=0  x0=0  Ts=activePowerSampleTime
  Low-Pass Filter (Discrete or Continuous) : eeGeneralControl/Low-Pass Filter (Discrete or Continuous)  K=1  T=vsmPmeasFilterTC  B=inf  A=-inf  init_option=Specify as parameter  x0=0  Ts=activePowerSampleTime
  Power Reference Selection : Subsystem
  Saturation : Saturate  UpperLimit=dampingPowerMaxLimit  LowerLimit=dampingPowerMinLimit
  Scope : Scope
  Sum1 : Sum  Inputs=-+-|
  Sum2 : Sum  Inputs=|+-
  Unit Delay : UnitDelay  SampleTime=-1
  Unit Delay1 : UnitDelay  SampleTime=-1
  Theta : Outport
  w : Outport  Port=2
  wires:
  Integrator with Wrapped State (Discrete or Continuous)/1 -> Add/1
  Sum1/1 -> Gain1/1  "Pinertia"
  Constant2/1 -> Add/2
  Add/1 -> Theta/1
  Discrete-Time Integrator/1 -> Gain/1, Unit Delay1/1, Sum2/1
  Low-Pass Filter (Discrete or Continuous)/1 -> Sum1/1
  Gain2/1 -> Saturation/1
  Power Reference Selection/1(power) -> Sum1/2
  Sum2/1 -> Unit Delay/1
  Gain1/1 -> Discrete-Time Integrator/1
  Gain/1 -> Integrator with Wrapped State (Discrete or Continuous)/1, Scope/1, w/1
  Unit Delay/1 -> Gain2/1
  Unit Delay1/1 -> [Wsm]
  Saturation/1 -> Sum1/3  "Pdamping"
  fgrid/1 -> Damping Frequency/1(fref)
  Damping Frequency/1(fmeas) -> Sum2/2
  cntrlflag/1 -> Power Reference Selection/1(cntrlflag)
  Pref/1 -> Power Reference Selection/2(Pref)
  fref/1 -> Power Reference Selection/3(fref)
  Pmeas/1 -> Low-Pass Filter (Discrete or Continuous)/1
  [Wsm] -> Power Reference Selection/4(Wsm)

== system SimscapeCustomComponents_lib/Microgrid and Renewables/Control/BESS/Grid Forming Control/Power Control/ReactiveControl/Voltage  Reference Selection ==
  cntrlflag : Inport
  Qref : Inport  Port=2
  Qmeas : Inport  Port=3
  Vref : Inport  Port=4
  Vgdmeas : Inport  Port=5
  If : If
  If Action Subsystem : Subsystem  TreatAsAtomicUnit=on
  If Action Subsystem1 : Subsystem  TreatAsAtomicUnit=on
  Merge : Merge
  Rate Transition : RateTransition
  Vd : Outport
  wires:
  If/1 -> If Action Subsystem/Action
  If Action Subsystem/1(Vd) -> Merge/1
  If/2 -> If Action Subsystem1/Action
  cntrlflag/1 -> Rate Transition/1
  Merge/1 -> Vd/1
  Qmeas/1 -> If Action Subsystem/2(Qmeas)
  Qref/1 -> If Action Subsystem/1(Qref)
  If Action Subsystem1/1(Voltage) -> Merge/2
  Vref/1 -> If Action Subsystem1/1(Vref)
  Vgdmeas/1 -> If Action Subsystem1/2(Vmeas)
  Rate Transition/1 -> If/1

== system SimscapeCustomComponents_lib/Microgrid and Renewables/Control/BESS/Grid Forming Control/VoltageCurrentControl/Controller/Id Current Limiting ==
  Imax : Inport
  Id : Inport  Port=2
  Abs : Abs  SaturateOnIntegerOverflow=off
  Switch : Switch  Criteria=u2 > Threshold  SaturateOnIntegerOverflow=off  InputSameDT=off
  Idref : Outport
  wires:
  Id/1 -> Switch/3
  Abs/1 -> Switch/2
  Imax/1 -> Abs/1, Switch/1
  Switch/1 -> Idref/1

== system SimscapeCustomComponents_lib/Microgrid and Renewables/Control/BESS/Grid Forming Control/VoltageCurrentControl/Controller/Iq Current Limiting ==
  Imax : Inport
  Iq : Inport  Port=2
  Abs : Abs  SaturateOnIntegerOverflow=off
  Switch : Switch  Criteria=u2 > Threshold  SaturateOnIntegerOverflow=off  InputSameDT=off
  Iqref : Outport
  wires:
  Iq/1 -> Switch/3
  Abs/1 -> Switch/2
  Imax/1 -> Abs/1, Switch/1
  Switch/1 -> Iqref/1
